simulink model "Demo1_P1A4"  (R2023a)
settings: Solver=VariableStepAuto  StartTime=0.0  StopTime=10.0  RelTol=1e-3
settings Model: Creator=rqouta  LastModifiedBy=rqouta

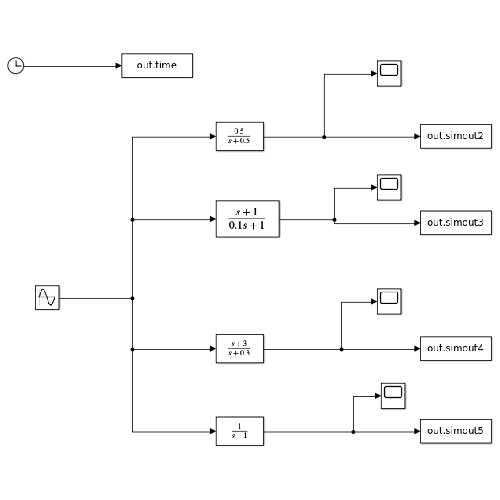
[thumbnail: Simulink's stored preview of the top-level diagram]
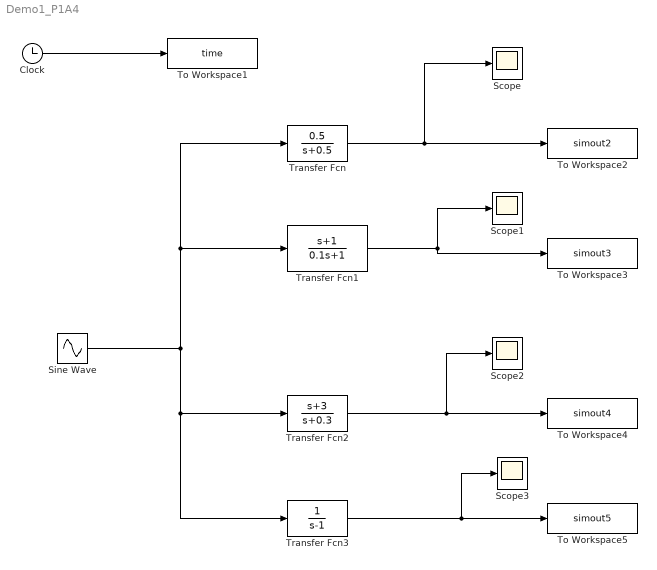
== system Demo1_P1A4 ==
  Clock : Clock
  Scope{,1..3} (4 alike) : Scope
  Sine Wave : Sin  SampleTime=0
  To Workspace1 : ToWorkspace  VariableName=time  SampleTime=-1
  To Workspace2 : ToWorkspace  VariableName=simout2  SampleTime=-1
  To Workspace3 : ToWorkspace  VariableName=simout3  SampleTime=-1
  To Workspace4 : ToWorkspace  VariableName=simout4  SampleTime=-1
  To Workspace5 : ToWorkspace  VariableName=simout5  SampleTime=-1
  Transfer Fcn : TransferFcn  Numerator=[0.5]  Denominator=[1 0.5]
  Transfer Fcn1 : TransferFcn  Numerator=[1 1]  Denominator=[0.1 1]
  Transfer Fcn2 : TransferFcn  Numerator=[1 3]  Denominator=[1 0.3]
  Transfer Fcn3 : TransferFcn  Denominator=[1 -1]
  wires:
  Clock/1 -> To Workspace1/1
  Sine Wave/1 -> Transfer Fcn3/1, Transfer Fcn2/1, Transfer Fcn1/1, Transfer Fcn/1
  Transfer Fcn2/1 -> Scope2/1, To Workspace4/1
  Transfer Fcn/1 -> Scope/1, To Workspace2/1
  Transfer Fcn1/1 -> To Workspace3/1, Scope1/1
  Transfer Fcn3/1 -> Scope3/1, To Workspace5/1
